simulink model "exp_asynchronous_model"  (R2020a)
settings: Solver=ode5  StartTime=0.0  StopTime=60  FixedStep=sampTime  RelTol=1e-3
values from neighbouring files (symbols this model uses):
  cutoffRad = 100*2*pi    (= 628.318530718)    [exp_asynchronous_script.m]
  encCPR = 4096    [exp_asynchronous_script.m]
  imp_dur = 0.02    [exp_asynchronous_script.m]
  imp_mag = 1    [exp_asynchronous_script.m]
  imp_start = 0.5    [exp_asynchronous_script.m]
  SA_kernel = gain_scaling * gain_constant*(1-synch_gain_range(k)) * temp_kernel    [exp_asynchronous_script.m]
  sampTime = 0.001    [exp_asynchronous_script.m]
  synch_gain = synch_gain_range(k) * gain_constant    [exp_asynchronous_script.m]
  synch_w = synch_freq * 2 * pi    [exp_asynchronous_script.m]
undefined symbols (not defined in the file or in its folder): National_Instruments, PCIe, Serial_Port, Standard_Devices
libraries: sldrtlib x2, cstblocks x1
settings Model: SimulationMode=external  ExtModeTrigDuration=500000  Creator=Gravish Lab  LastModifiedBy=Gravish Lab
settings DataIOCC: ReturnWorkspaceOutputs=off
settings RTWCC: Description=Simulink Desktop Real-Time  SystemTargetFile=sldrt.tlc  TemplateMakefile=sldrt.tmf  RTWCompilerOptimization=on
settings CodeAppCC: MaxIdLength=95
settings SimulinkDesktopRealTimeCC: TargetPreCompLibLocation=C:\Program Files\MATLAB\R2020a\toolbox\sldrt\lib\win64

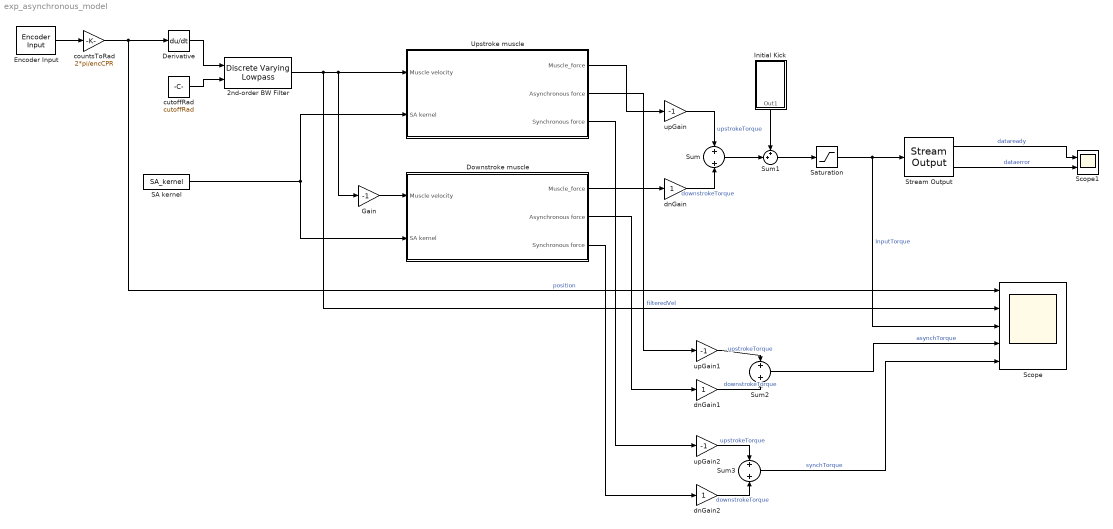
== system exp_asynchronous_model ==
  2nd-order BW Filter : cstblocks/Linear Parameter Varying/Discrete Varying Lowpass  N=2  w0=0  Ts=sampTime
      settings: SourceProductBaseCode=CT
  Derivative : Derivative
  Downstroke muscle : Subsystem
  Encoder Input : sldrtlib/Encoder Input  SampleTime=sampTime  MaxMissedTicks=1000  ShowMissedTicks=off  YieldWhenWaiting=on  DrvName=National_Instruments/PCIe-6323  DrvAddress=4294967295  DrvOptions=[0 0 0 3 0 2 2]  Channels=4  QuadMode=3  IndexPulse=1  InputFilter=Inf  DataType=1
      settings: AttributesFormatString=National Instruments\nPCIe-6323 [auto]
  Gain : Gain  Gain=-1
  Initial Kick : Subsystem
  SA kernel : Constant  Value=SA_kernel
  Saturation : Saturate  UpperLimit=4  LowerLimit=-4
  Scope : Scope  NumInputPorts=5
  Scope1 : Scope  NumInputPorts=2
  Stream Output : sldrtlib/Stream Output  SampleTime=0.001  MaxMissedTicks=10  ShowMissedTicks=off  YieldWhenWaiting=on  DrvName=Standard_Devices/Serial_Port  DrvAddress=5  DrvOptions=[115200 8 0 0 0 0 0 0]  PortSizes=1  FormatString='w axis0.controller.input_torque %1.3f\n'  ShowReady=on  ShowError=on  InitialValue='w axis0.controller.input_torque 0\n'  FinalValue='w axis0.controller.input_torque 0\n'
      settings: AttributesFormatString=Serial Port [5]  SourceProductBaseCode=WT
  Sum : Sum  Inputs=+|+
  Sum1 : Sum  Inputs=++|
  Sum2 : Sum  Inputs=+|+
  Sum3 : Sum  Inputs=+|+
  Upstroke muscle : Subsystem
  countsToRad : Gain  Gain=2*pi/encCPR
  cutoffRad : Constant  Value=cutoffRad
  dnGain : Gain
  dnGain1 : Gain
  dnGain2 : Gain
  upGain : Gain  Gain=-1
  upGain1 : Gain  Gain=-1
  upGain2 : Gain  Gain=-1
  wires:
  Encoder Input/1 -> countsToRad/1
  countsToRad/1 -> Scope/1, Derivative/1  "position"
  Gain/1 -> Downstroke muscle/1(Muscle velocity)
  SA kernel/1 -> Downstroke muscle/2(SA kernel), Upstroke muscle/2(SA kernel)
  Upstroke muscle/1(Muscle_force) -> upGain/1
  upGain/1 -> Sum/1  "upstrokeTorque"
  dnGain/1 -> Sum/2  "downstrokeTorque"
  Sum/1 -> Sum1/2
  Initial Kick/1(Out1) -> Sum1/1
  Derivative/1 -> 2nd-order BW Filter/1
  cutoffRad/1 -> 2nd-order BW Filter/2
  2nd-order BW Filter/1 -> Scope/2, Upstroke muscle/1(Muscle velocity), Gain/1  "filteredVel"
  Downstroke muscle/1(Muscle_force) -> dnGain/1
  Saturation/1 -> Stream Output/1, Scope/3  "InputTorque"
  Sum1/1 -> Saturation/1
  Upstroke muscle/2(Asynchronous force) -> upGain1/1
  Downstroke muscle/2(Asynchronous force) -> dnGain1/1
  Upstroke muscle/3(Synchronous force) -> upGain2/1
  Downstroke muscle/3(Synchronous force) -> dnGain2/1
  upGain1/1 -> Sum2/1  "upstrokeTorque"
  dnGain1/1 -> Sum2/2  "downstrokeTorque"
  upGain2/1 -> Sum3/1  "upstrokeTorque"
  dnGain2/1 -> Sum3/2  "downstrokeTorque"
  Sum2/1 -> Scope/4  "asynchTorque"
  Sum3/1 -> Scope/5  "synchTorque"
  Stream Output/1 -> Scope1/1  "dataready"
  Stream Output/2 -> Scope1/2  "dataerror"

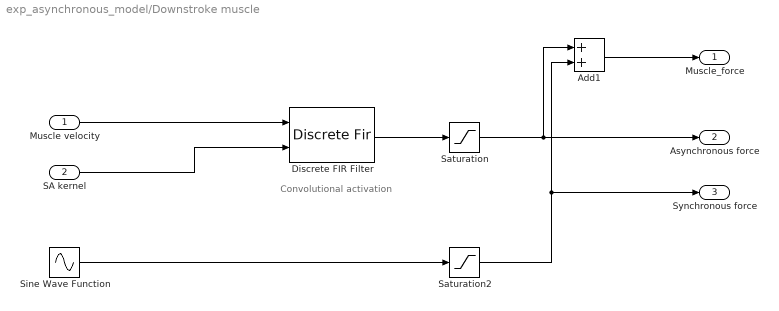
== system exp_asynchronous_model/Downstroke muscle ==
  note: Convolutional activation
  Muscle velocity : Inport
  SA kernel : Inport  Port=2
  Add1 : Sum
  Discrete FIR Filter : DiscreteFir  CoefSource=Input port  Coefficients=[0, 0, 2]  InputProcessing=Columns as channels (frame based)
      settings: InputPortMap=u0,u1
  Saturation : Saturate  UpperLimit=Inf  LowerLimit=0
  Saturation2 : Saturate  UpperLimit=Inf  LowerLimit=0
  Sine Wave Function : Sin  Amplitude=synch_gain  Frequency=synch_w  Phase=pi  SampleTime=0
  Muscle_force : Outport
  Asynchronous force : Outport  Port=2
  Synchronous force : Outport  Port=3
  wires:
  Saturation/1 -> Asynchronous force/1, Add1/1
  SA kernel/1 -> Discrete FIR Filter/2
  Add1/1 -> Muscle_force/1
  Discrete FIR Filter/1 -> Saturation/1
  Sine Wave Function/1 -> Saturation2/1
  Saturation2/1 -> Synchronous force/1, Add1/2
  Muscle velocity/1 -> Discrete FIR Filter/1

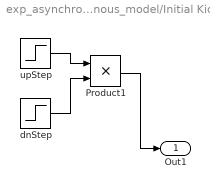
== system exp_asynchronous_model/Initial Kick ==
  Product1 : Product
  dnStep : Step  Time=imp_start+imp_dur  Before=1  After=0  SampleTime=0
  upStep : Step  Time=imp_start  After=imp_mag  SampleTime=0
  Out1 : Outport
  wires:
  Product1/1 -> Out1/1
  dnStep/1 -> Product1/2
  upStep/1 -> Product1/1

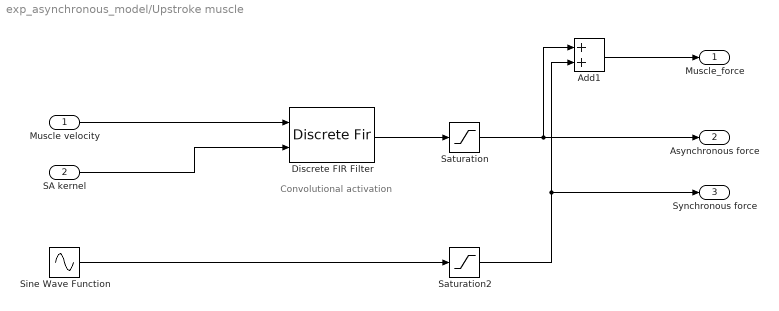
== system exp_asynchronous_model/Upstroke muscle ==
  note: Convolutional activation
  Muscle velocity : Inport
  SA kernel : Inport  Port=2
  Add1 : Sum
  Discrete FIR Filter : DiscreteFir  CoefSource=Input port  Coefficients=[0, 0, 2]  InputProcessing=Columns as channels (frame based)
      settings: InputPortMap=u0,u1
  Saturation : Saturate  UpperLimit=Inf  LowerLimit=0
  Saturation2 : Saturate  UpperLimit=Inf  LowerLimit=0
  Sine Wave Function : Sin  Amplitude=synch_gain  Frequency=synch_w  SampleTime=0
  Muscle_force : Outport
  Asynchronous force : Outport  Port=2
  Synchronous force : Outport  Port=3
  wires:
  Saturation/1 -> Asynchronous force/1, Add1/1
  SA kernel/1 -> Discrete FIR Filter/2
  Add1/1 -> Muscle_force/1
  Discrete FIR Filter/1 -> Saturation/1
  Sine Wave Function/1 -> Saturation2/1
  Saturation2/1 -> Synchronous force/1, Add1/2
  Muscle velocity/1 -> Discrete FIR Filter/1
